simulink model "nmn (2)"  (R2018a)
settings: Solver=VariableStepAuto  StartTime=0.0  StopTime=6  RelTol=1e-3
values from neighbouring files (symbols this model uses):
  A = diag([-1,-2,-3,-4,-5])    [HW2_2.m]    (also in N1.m = [0 0 1 0; 0 0 0 1; -0.4568 -0.6196 0 0;0.2485 -6.6174 0 0]; N19.m = [0 0 1 0; 0 0 0 1; -0.4568 -0.6196 0 0;0.2485 -6.6174 0 0]; Q24.m = [0 1;0 0]; Q36.m = [a11 a12 0 -g;a21 a22 1 0;a31 a31 a33 0;0 1 0 0])
  A_n = A-L*C    [N19.m]
  B = [0 0; 0 0; 0.7870 -0.0426; 0.0426 0.1349]    [N1.m]    (also in N19.m; Q24.m = [0 1]'; Q36.m = [b1;b2;b3;0]; Q41.m = [0;-0.036;-12.61;0])
  B_n = B    [N19.m]
  C = [1 0 0 0; 0 1 0 0]    [N1.m]    (also in N19.m; Q21.m = ctrb; Q24.m = [1 0;0 1]; Q36.m = [1 0 0 0])
  C_n = C    [N19.m]
  L = (place(A',C',Pole_r))'    [N19.m]    (also in Q41.m = [L_taw [0 1;1 0]])
libraries: simulink x1
settings Model: Creator=m  LastModifiedBy=m

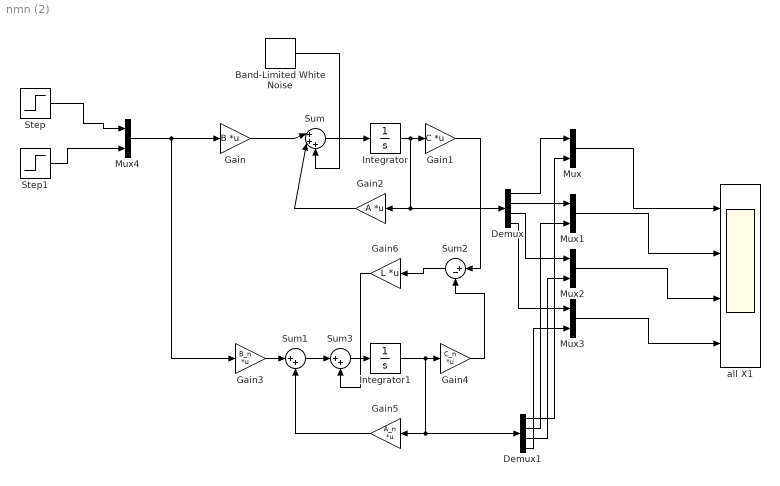
== system nmn (2) ==
  Band-Limited White Noise : simulink/Sources/Band-Limited White Noise  Cov=[0.01]  Ts=0.8  seed=[23341]
  Demux : Demux
  Demux1 : Demux
  Gain : Gain  Gain=B  Multiplication=Matrix(K*u) (u vector)
  Gain1 : Gain  Gain=C  Multiplication=Matrix(K*u) (u vector)
  Gain2 : Gain  Gain=A  Multiplication=Matrix(K*u) (u vector)
  Gain3 : Gain  Gain=B_n  Multiplication=Matrix(K*u) (u vector)
  Gain4 : Gain  Gain=C_n  Multiplication=Matrix(K*u) (u vector)
  Gain5 : Gain  Gain=A_n  Multiplication=Matrix(K*u) (u vector)
  Gain6 : Gain  Gain=L  Multiplication=Matrix(K*u) (u vector)
  Integrator : Integrator
  Integrator1 : Integrator
  Mux{,1..4} (5 alike) : Mux  Inputs=2
  Step : Step  Time=0  SampleTime=0
  Step1 : Step  Time=0  SampleTime=0
  Sum : Sum  Inputs=|+++
  Sum1 : Sum  Inputs=|++
  Sum2 : Sum  Inputs=|+-
  Sum3 : Sum  Inputs=|++
  all X1 : Scope  NumInputPorts=4
  wires:
  Step/1 -> Mux4/1
  Step1/1 -> Mux4/2
  Gain/1 -> Sum/1
  Gain2/1 -> Sum/2
  Sum/1 -> Integrator/1
  Integrator/1 -> Gain1/1, Gain2/1, Demux/1
  Mux4/1 -> Gain/1, Gain3/1
  Integrator1/1 -> Gain5/1, Demux1/1, Gain4/1
  Demux/1 -> Mux/1
  Demux1/1 -> Mux/2
  Mux/1 -> all X1/1
  Demux/2 -> Mux1/1
  Demux1/2 -> Mux1/2
  Demux1/3 -> Mux2/2
  Demux/3 -> Mux2/1
  Demux/4 -> Mux3/1
  Demux1/4 -> Mux3/2
  Mux1/1 -> all X1/2
  Mux2/1 -> all X1/3
  Mux3/1 -> all X1/4
  Gain4/1 -> Sum2/2
  Gain1/1 -> Sum2/1
  Sum2/1 -> Gain6/1
  Gain3/1 -> Sum1/1
  Gain5/1 -> Sum1/2
  Sum1/1 -> Sum3/1
  Gain6/1 -> Sum3/2
  Sum3/1 -> Integrator1/1
  Band-Limited White Noise/1 -> Sum/3
